simulink model "LUT_kidney_25"  (R2023b)
settings: Solver=FixedStepAuto  StartTime=0  StopTime=10.1  FixedStep=Timegap  RelTol=1e-3
model workspace (MAT data in the model file):
  T1_input = 1.34
(part 2 of 3)

== system LUT_kidney_25/If Action Subsystem6/If Action Subsystem1/If Action Subsystem6/If Action Subsystem4 ==
  In1 : Inport
  Action Port : ActionPort  ActionPortLabel=elseif( u1 >= 1.035)
  LUT 1.04RR : Lookup_n-D  NumberOfTableDimensions=1  BreakpointsForDimension1=[434.5226;535.5743;634.3365;733.4874;832.6376;931.7698;1030.887;1129.994;1229.093;1328.188;1427.279;1526.369;1625.457;1724.544;1823.63;1922.716;2021.797]  Table=[400;500;600;700;800;900;1000;1100;1200;1300;1400;1500;1600;1700;1800;1900;2000]  InternalRulePriority=Speed  RndMeth=Simplest
  Out1 : Outport
  wires:
  In1/1 -> LUT 1.04RR/1
  LUT 1.04RR/1 -> Out1/1

== system LUT_kidney_25/If Action Subsystem6/If Action Subsystem1/If Action Subsystem6/If Action Subsystem5 ==
  In1 : Inport
  Action Port : ActionPort  ActionPortLabel=elseif( u1 >= 1.055)
  LUT 1.06RR : Lookup_n-D  NumberOfTableDimensions=1  BreakpointsForDimension1=[434.2491;535.1556;633.7517;732.7193;831.6764;930.6091;1029.523;1128.423;1227.313;1326.197;1425.077;1523.953;1622.827;1721.7;1820.571;1919.441;2018.308]  Table=[400;500;600;700;800;900;1000;1100;1200;1300;1400;1500;1600;1700;1800;1900;2000]  InternalRulePriority=Speed  RndMeth=Simplest
  Out1 : Outport
  wires:
  In1/1 -> LUT 1.06RR/1
  LUT 1.06RR/1 -> Out1/1

== system LUT_kidney_25/If Action Subsystem6/If Action Subsystem1/If Action Subsystem6/If Action Subsystem6 ==
  In1 : Inport
  Action Port : ActionPort  ActionPortLabel=elseif( u1 >= 1.045)
  LUT 1.05RR : Lookup_n-D  NumberOfTableDimensions=1  BreakpointsForDimension1=[434.3843;535.3623;634.0403;733.0983;832.1508;931.1821;1030.196;1129.199;1228.192;1327.181;1426.165;1525.147;1624.126;1723.105;1822.083;1921.059;2020.032]  Table=[400;500;600;700;800;900;1000;1100;1200;1300;1400;1500;1600;1700;1800;1900;2000]  InternalRulePriority=Speed  RndMeth=Simplest
  Out1 : Outport
  wires:
  In1/1 -> LUT 1.05RR/1
  LUT 1.05RR/1 -> Out1/1

== system LUT_kidney_25/If Action Subsystem6/If Action Subsystem1/If Action Subsystem6/If Action Subsystem7 ==
  In1 : Inport
  Action Port : ActionPort  ActionPortLabel=elseif( u1 >= 1.065)
  LUT 1.07RR : Lookup_n-D  NumberOfTableDimensions=1  BreakpointsForDimension1=[434.1166;534.9541;633.4706;732.35;831.2139;930.0504;1028.866;1127.666;1226.455;1325.237;1424.014;1522.787;1621.558;1720.327;1819.094;1917.859;2016.622]  Table=[400;500;600;700;800;900;1000;1100;1200;1300;1400;1500;1600;1700;1800;1900;2000]  InternalRulePriority=Speed  RndMeth=Simplest
  Out1 : Outport
  wires:
  In1/1 -> LUT 1.07RR/1
  LUT 1.07RR/1 -> Out1/1

== system LUT_kidney_25/If Action Subsystem6/If Action Subsystem1/If Action Subsystem6/If Action Subsystem8 ==
  In1 : Inport
  Action Port : ActionPort  ActionPortLabel=elseif(u1 >= 1.075)
  LUT 1.08RR : Lookup_n-D  NumberOfTableDimensions=1  BreakpointsForDimension1=[433.987;534.7575;633.1966;731.9901;830.763;929.5054;1028.224;1126.927;1225.617;1324.299;1422.976;1521.648;1620.317;1718.984;1817.65;1916.313;2014.973]  Table=[400;500;600;700;800;900;1000;1100;1200;1300;1400;1500;1600;1700;1800;1900;2000]  InternalRulePriority=Speed  RndMeth=Simplest
  Out1 : Outport
  wires:
  In1/1 -> LUT 1.08RR/1
  LUT 1.08RR/1 -> Out1/1

== system LUT_kidney_25/If Action Subsystem6/If Action Subsystem1/If Action Subsystem6/If Action Subsystem9 ==
  In1 : Inport
  Action Port : ActionPort  ActionPortLabel=if(u1 >= 1.085)
  LUT 1.09RR : Lookup_n-D  NumberOfTableDimensions=1  BreakpointsForDimension1=[433.8599;534.5681;632.9294;731.6391;830.3233;928.9736;1027.598;1126.205;1224.799;1323.383;1421.962;1520.535;1619.105;1717.672;1816.237;1914.801;2013.361]  Table=[400;500;600;700;800;900;1000;1100;1200;1300;1400;1500;1600;1700;1800;1900;2000]  InternalRulePriority=Speed  RndMeth=Simplest
  Out1 : Outport
  wires:
  In1/1 -> LUT 1.09RR/1
  LUT 1.09RR/1 -> Out1/1

== system LUT_kidney_25/If Action Subsystem6/If Action Subsystem1/If Action Subsystem7/If Action Subsystem1 ==
  In1 : Inport
  Action Port : ActionPort  ActionPortLabel=elseif( u1 >= 1.215)
  LUT 1.22RR : Lookup_n-D  NumberOfTableDimensions=1  BreakpointsForDimension1=[432.4057;532.4278;629.9781;727.7664;825.4645;923.086;1020.653;1118.181;1215.681;1313.16;1410.624;1508.077;1605.521;1702.957;1800.388;1897.814;1995.235]  Table=[400;500;600;700;800;900;1000;1100;1200;1300;1400;1500;1600;1700;1800;1900;2000]  InternalRulePriority=Speed  RndMeth=Simplest
  Out1 : Outport
  wires:
  In1/1 -> LUT 1.22RR/1
  LUT 1.22RR/1 -> Out1/1

== system LUT_kidney_25/If Action Subsystem6/If Action Subsystem1/If Action Subsystem7/If Action Subsystem10 ==
  In1 : Inport
  Action Port : ActionPort  ActionPortLabel=elseif( u1 >= 1.205)
  LUT 1.21RR : Lookup_n-D  NumberOfTableDimensions=1  BreakpointsForDimension1=[432.5065;532.5721;630.1754;728.0248;825.789;923.48;1021.118;1118.72;1216.294;1313.849;1411.39;1508.919;1606.44;1703.953;1801.462;1898.966;1996.466]  Table=[400;500;600;700;800;900;1000;1100;1200;1300;1400;1500;1600;1700;1800;1900;2000]  InternalRulePriority=Speed  RndMeth=Simplest
  Out1 : Outport
  wires:
  In1/1 -> LUT 1.21RR/1
  LUT 1.21RR/1 -> Out1/1

== system LUT_kidney_25/If Action Subsystem6/If Action Subsystem1/If Action Subsystem7/If Action Subsystem2 ==
  In1 : Inport
  Action Port : ActionPort  ActionPortLabel=else
  LUT 1.20RR : Lookup_n-D  NumberOfTableDimensions=1  BreakpointsForDimension1=[432.6089;532.7193;630.3771;728.2891;826.1208;923.8827;1021.594;1119.27;1216.921;1314.553;1412.171;1509.778;1607.377;1704.97;1802.558;1900.141;1997.72]  Table=[400;500;600;700;800;900;1000;1100;1200;1300;1400;1500;1600;1700;1800;1900;2000]  InternalRulePriority=Speed  RndMeth=Simplest
  Out1 : Outport
  wires:
  In1/1 -> LUT 1.20RR/1
  LUT 1.20RR/1 -> Out1/1

== system LUT_kidney_25/If Action Subsystem6/If Action Subsystem1/If Action Subsystem7/If Action Subsystem3 ==
  In1 : Inport
  Action Port : ActionPort  ActionPortLabel=elseif( u1 >= 1.225)
  LUT 1.23RR : Lookup_n-D  NumberOfTableDimensions=1  BreakpointsForDimension1=[432.3064;532.2863;629.7849;727.5136;825.147;922.7006;1020.197;1117.653;1215.08;1312.485;1409.875;1507.252;1604.62;1701.98;1799.335;1896.684;1994.029]  Table=[400;500;600;700;800;900;1000;1100;1200;1300;1400;1500;1600;1700;1800;1900;2000]  InternalRulePriority=Speed  RndMeth=Simplest
  Out1 : Outport
  wires:
  In1/1 -> LUT 1.23RR/1
  LUT 1.23RR/1 -> Out1/1

== system LUT_kidney_25/If Action Subsystem6/If Action Subsystem1/If Action Subsystem7/If Action Subsystem4 ==
  In1 : Inport
  Action Port : ActionPort  ActionPortLabel=elseif( u1 >= 1.235)
  LUT 1.24RR : Lookup_n-D  NumberOfTableDimensions=1  BreakpointsForDimension1=[432.2086;532.1477;629.596;727.2663;824.8365;922.3235;1019.751;1117.136;1214.492;1311.824;1409.14;1506.444;1603.737;1701.023;1798.302;1895.576;1992.846]  Table=[400;500;600;700;800;900;1000;1100;1200;1300;1400;1500;1600;1700;1800;1900;2000]  InternalRulePriority=Speed  RndMeth=Simplest
  Out1 : Outport
  wires:
  In1/1 -> LUT 1.24RR/1
  LUT 1.24RR/1 -> Out1/1

== system LUT_kidney_25/If Action Subsystem6/If Action Subsystem1/If Action Subsystem7/If Action Subsystem5 ==
  In1 : Inport
  Action Port : ActionPort  ActionPortLabel=elseif( u1 >= 1.255)
  LUT 1.26RR : Lookup_n-D  NumberOfTableDimensions=1  BreakpointsForDimension1=[432.0174;531.8783;629.2298;726.7877;824.2353;921.5931;1018.887;1116.135;1213.351;1310.542;1407.715;1504.875;1602.023;1699.163;1796.297;1893.424;1990.547]  Table=[400;500;600;700;800;900;1000;1100;1200;1300;1400;1500;1600;1700;1800;1900;2000]  InternalRulePriority=Speed  RndMeth=Simplest
  Out1 : Outport
  wires:
  In1/1 -> LUT 1.26RR/1
  LUT 1.26RR/1 -> Out1/1

== system LUT_kidney_25/If Action Subsystem6/If Action Subsystem1/If Action Subsystem7/If Action Subsystem6 ==
  In1 : Inport
  Action Port : ActionPort  ActionPortLabel=elseif( u1 >= 1.245)
  LUT 1.25RR : Lookup_n-D  NumberOfTableDimensions=1  BreakpointsForDimension1=[432.1123;532.0117;629.411;727.0244;824.5326;921.9544;1019.314;1116.631;1213.915;1311.177;1408.421;1505.651;1602.872;1700.084;1797.29;1894.49;1991.685]  Table=[400;500;600;700;800;900;1000;1100;1200;1300;1400;1500;1600;1700;1800;1900;2000]  InternalRulePriority=Speed  RndMeth=Simplest
  Out1 : Outport
  wires:
  In1/1 -> LUT 1.25RR/1
  LUT 1.25RR/1 -> Out1/1

== system LUT_kidney_25/If Action Subsystem6/If Action Subsystem1/If Action Subsystem7/If Action Subsystem7 ==
  In1 : Inport
  Action Port : ActionPort  ActionPortLabel=elseif( u1 >= 1.265)
  LUT 1.27RR : Lookup_n-D  NumberOfTableDimensions=1  BreakpointsForDimension1=[431.9239;531.7475;629.0525;726.556;823.9443;921.2395;1018.468;1115.65;1212.798;1309.92;1407.024;1504.113;1601.191;1698.26;1795.322;1892.379;1989.43]  Table=[400;500;600;700;800;900;1000;1100;1200;1300;1400;1500;1600;1700;1800;1900;2000]  InternalRulePriority=Speed  RndMeth=Simplest
  Out1 : Outport
  wires:
  In1/1 -> LUT 1.27RR/1
  LUT 1.27RR/1 -> Out1/1

== system LUT_kidney_25/If Action Subsystem6/If Action Subsystem1/If Action Subsystem7/If Action Subsystem8 ==
  In1 : Inport
  Action Port : ActionPort  ActionPortLabel=elseif(u1 >= 1.275)
  LUT 1.28RR : Lookup_n-D  NumberOfTableDimensions=1  BreakpointsForDimension1=[431.8317;531.6191;628.8788;726.3292;823.6595;920.8933;1018.058;1115.175;1212.256;1309.311;1406.346;1503.366;1600.375;1697.375;1794.367;1891.353;1988.334]  Table=[400;500;600;700;800;900;1000;1100;1200;1300;1400;1500;1600;1700;1800;1900;2000]  InternalRulePriority=Speed  RndMeth=Simplest
  Out1 : Outport
  wires:
  In1/1 -> LUT 1.28RR/1
  LUT 1.28RR/1 -> Out1/1

== system LUT_kidney_25/If Action Subsystem6/If Action Subsystem1/If Action Subsystem7/If Action Subsystem9 ==
  In1 : Inport
  Action Port : ActionPort  ActionPortLabel=if(u1 >= 1.285)
  LUT 1.29RR : Lookup_n-D  NumberOfTableDimensions=1  BreakpointsForDimension1=[431.7409;531.4931;628.7087;726.1072;823.3807;920.5544;1017.657;1114.709;1211.725;1308.713;1405.681;1502.634;1599.575;1696.506;1793.429;1890.346;1987.258]  Table=[400;500;600;700;800;900;1000;1100;1200;1300;1400;1500;1600;1700;1800;1900;2000]  InternalRulePriority=Speed  RndMeth=Simplest
  Out1 : Outport
  wires:
  In1/1 -> LUT 1.29RR/1
  LUT 1.29RR/1 -> Out1/1

== system LUT_kidney_25/If Action Subsystem6/If Action Subsystem1/If Action Subsystem8/If Action Subsystem1 ==
  In1 : Inport
  Action Port : ActionPort  ActionPortLabel=elseif( u1 >= 1.315)
  LUT 1.32RR : Lookup_n-D  NumberOfTableDimensions=1  BreakpointsForDimension1=[431.4756;531.1287;628.2187;725.4687;822.5789;919.5791;1016.501;1113.368;1210.194;1306.99;1403.764;1500.521;1597.264;1693.997;1790.721;1887.438;1984.149]  Table=[400;500;600;700;800;900;1000;1100;1200;1300;1400;1500;1600;1700;1800;1900;2000]  InternalRulePriority=Speed  RndMeth=Simplest
  Out1 : Outport
  wires:
  In1/1 -> LUT 1.32RR/1
  LUT 1.32RR/1 -> Out1/1

== system LUT_kidney_25/If Action Subsystem6/If Action Subsystem1/If Action Subsystem8/If Action Subsystem10 ==
  In1 : Inport
  Action Port : ActionPort  ActionPortLabel=elseif( u1 >= 1.305)
  LUT 1.31RR : Lookup_n-D  NumberOfTableDimensions=1  BreakpointsForDimension1=[431.5628;531.248;628.3787;725.6771;822.8406;919.8974;1016.879;1113.806;1210.694;1307.553;1404.391;1501.212;1598.02;1694.817;1791.607;1888.389;1985.166]  Table=[400;500;600;700;800;900;1000;1100;1200;1300;1400;1500;1600;1700;1800;1900;2000]  InternalRulePriority=Speed  RndMeth=Simplest
  Out1 : Outport
  wires:
  In1/1 -> LUT 1.31RR/1
  LUT 1.31RR/1 -> Out1/1

== system LUT_kidney_25/If Action Subsystem6/If Action Subsystem1/If Action Subsystem8/If Action Subsystem2 ==
  In1 : Inport
  Action Port : ActionPort  ActionPortLabel=else
  LUT 1.30RR : Lookup_n-D  NumberOfTableDimensions=1  BreakpointsForDimension1=[431.6512;531.3694;628.542;725.8899;823.1078;920.2225;1017.264;1114.253;1211.204;1308.127;1405.03;1501.916;1598.79;1695.654;1792.509;1889.359;1986.202]  Table=[400;500;600;700;800;900;1000;1100;1200;1300;1400;1500;1600;1700;1800;1900;2000]  InternalRulePriority=Speed  RndMeth=Simplest
  Out1 : Outport
  wires:
  In1/1 -> LUT 1.30RR/1
  LUT 1.30RR/1 -> Out1/1

== system LUT_kidney_25/If Action Subsystem6/If Action Subsystem1/If Action Subsystem8/If Action Subsystem3 ==
  In1 : Inport
  Action Port : ActionPort  ActionPortLabel=elseif( u1 >= 1.325)
  LUT 1.33RR : Lookup_n-D  NumberOfTableDimensions=1  BreakpointsForDimension1=[431.3895;531.0116;628.0619;725.2646;822.3226;919.2673;1016.131;1112.938;1209.703;1306.438;1403.149;1499.843;1596.523;1693.191;1789.851;1886.503;1983.15]  Table=[400;500;600;700;800;900;1000;1100;1200;1300;1400;1500;1600;1700;1800;1900;2000]  InternalRulePriority=Speed  RndMeth=Simplest
  Out1 : Outport
  wires:
  In1/1 -> LUT 1.33RR/1
  LUT 1.33RR/1 -> Out1/1

== system LUT_kidney_25/If Action Subsystem6/If Action Subsystem1/If Action Subsystem8/If Action Subsystem4 ==
  In1 : Inport
  Action Port : ActionPort  ActionPortLabel=elseif( u1 >= 1.335)
  LUT 1.34RR : Lookup_n-D  NumberOfTableDimensions=1  BreakpointsForDimension1=[431.3046;530.8966;627.9082;725.0647;822.0716;918.9618;1015.769;1112.517;1209.223;1305.897;1402.546;1499.178;1595.795;1692.401;1788.997;1885.586;1982.169]  Table=[400;500;600;700;800;900;1000;1100;1200;1300;1400;1500;1600;1700;1800;1900;2000]  InternalRulePriority=Speed  RndMeth=Simplest
  Out1 : Outport
  wires:
  In1/1 -> LUT 1.34RR/1
  LUT 1.34RR/1 -> Out1/1

== system LUT_kidney_25/If Action Subsystem6/If Action Subsystem1/If Action Subsystem8/If Action Subsystem5 ==
  In1 : Inport
  Action Port : ActionPort  ActionPortLabel=elseif( u1 >= 1.355)
  LUT 1.36RR : Lookup_n-D  NumberOfTableDimensions=1  BreakpointsForDimension1=[431.138;530.6725;627.6097;724.6771;821.585;918.3694;1015.066;1111.7;1208.289;1304.845;1401.375;1497.885;1594.38;1690.863;1787.336;1883.801;1980.259]  Table=[400;500;600;700;800;900;1000;1100;1200;1300;1400;1500;1600;1700;1800;1900;2000]  InternalRulePriority=Speed  RndMeth=Simplest
  Out1 : Outport
  wires:
  In1/1 -> LUT 1.36RR/1
  LUT 1.36RR/1 -> Out1/1

== system LUT_kidney_25/If Action Subsystem6/If Action Subsystem1/If Action Subsystem8/If Action Subsystem6 ==
  In1 : Inport
  Action Port : ActionPort  ActionPortLabel=elseif( u1 >= 1.345)
  LUT 1.35RR : Lookup_n-D  NumberOfTableDimensions=1  BreakpointsForDimension1=[431.2207;530.7835;627.7575;724.8689;821.8258;918.6626;1015.414;1112.105;1208.752;1305.366;1401.955;1498.525;1595.081;1691.625;1788.159;1884.686;1981.205]  Table=[400;500;600;700;800;900;1000;1100;1200;1300;1400;1500;1600;1700;1800;1900;2000]  InternalRulePriority=Speed  RndMeth=Simplest
  Out1 : Outport
  wires:
  In1/1 -> LUT 1.35RR/1
  LUT 1.35RR/1 -> Out1/1

== system LUT_kidney_25/If Action Subsystem6/If Action Subsystem1/If Action Subsystem8/If Action Subsystem7 ==
  In1 : Inport
  Action Port : ActionPort  ActionPortLabel=elseif( u1 >= 1.365)
  LUT 1.37RR : Lookup_n-D  NumberOfTableDimensions=1  BreakpointsForDimension1=[431.0562;530.5633;627.4649;724.4891;821.3491;918.0821;1014.725;1111.304;1207.836;1304.334;1400.805;1497.256;1593.692;1690.115;1786.528;1882.932;1979.33]  Table=[400;500;600;700;800;900;1000;1100;1200;1300;1400;1500;1600;1700;1800;1900;2000]  InternalRulePriority=Speed  RndMeth=Simplest
  Out1 : Outport
  wires:
  In1/1 -> LUT 1.37RR/1
  LUT 1.37RR/1 -> Out1/1

== system LUT_kidney_25/If Action Subsystem6/If Action Subsystem1/If Action Subsystem8/If Action Subsystem8 ==
  In1 : Inport
  Action Port : ActionPort  ActionPortLabel=elseif(u1 >= 1.375)
  LUT 1.38RR : Lookup_n-D  NumberOfTableDimensions=1  BreakpointsForDimension1=[430.9755;530.4561;627.3228;724.305;821.1179;917.8006;1014.391;1110.915;1207.392;1303.832;1400.246;1496.64;1593.017;1689.381;1785.734;1882.079;1978.417]  Table=[400;500;600;700;800;900;1000;1100;1200;1300;1400;1500;1600;1700;1800;1900;2000]  InternalRulePriority=Speed  RndMeth=Simplest
  Out1 : Outport
  wires:
  In1/1 -> LUT 1.38RR/1
  LUT 1.38RR/1 -> Out1/1

== system LUT_kidney_25/If Action Subsystem6/If Action Subsystem1/If Action Subsystem8/If Action Subsystem9 ==
  In1 : Inport
  Action Port : ActionPort  ActionPortLabel=if(u1 >= 1.385)
  LUT 1.39RR : Lookup_n-D  NumberOfTableDimensions=1  BreakpointsForDimension1=[430.8958;530.3506;627.1835;724.1245;820.8914;917.5247;1014.063;1110.534;1206.956;1303.341;1399.698;1496.034;1592.353;1688.659;1784.955;1881.241;1977.521]  Table=[400;500;600;700;800;900;1000;1100;1200;1300;1400;1500;1600;1700;1800;1900;2000]  InternalRulePriority=Speed  RndMeth=Simplest
  Out1 : Outport
  wires:
  In1/1 -> LUT 1.39RR/1
  LUT 1.39RR/1 -> Out1/1

== system LUT_kidney_25/If Action Subsystem6/If Action Subsystem1/If Action Subsystem9/If Action Subsystem1 ==
  In1 : Inport
  Action Port : ActionPort  ActionPortLabel=elseif( u1 >= 1.415)
  LUT 1.42RR : Lookup_n-D  NumberOfTableDimensions=1  BreakpointsForDimension1=[430.6624;530.0447;626.7812;723.6044;820.2389;916.7296;1013.118;1109.434;1205.697;1301.92;1398.113;1494.283;1590.435;1686.572;1782.698;1878.814;1974.923]  Table=[400;500;600;700;800;900;1000;1100;1200;1300;1400;1500;1600;1700;1800;1900;2000]  InternalRulePriority=Speed  RndMeth=Simplest
  Out1 : Outport
  wires:
  In1/1 -> LUT 1.42RR/1
  LUT 1.42RR/1 -> Out1/1

== system LUT_kidney_25/If Action Subsystem6/If Action Subsystem1/If Action Subsystem9/If Action Subsystem10 ==
  In1 : Inport
  Action Port : ActionPort  ActionPortLabel=elseif( u1 >= 1.405)
  LUT 1.41RR : Lookup_n-D  NumberOfTableDimensions=1  BreakpointsForDimension1=[430.7393;530.1449;626.9128;723.7743;820.452;916.9894;1013.427;1109.794;1206.108;1302.384;1398.631;1494.856;1591.063;1687.256;1783.437;1879.609;1975.774]  Table=[400;500;600;700;800;900;1000;1100;1200;1300;1400;1500;1600;1700;1800;1900;2000]  InternalRulePriority=Speed  RndMeth=Simplest
  Out1 : Outport
  wires:
  In1/1 -> LUT 1.41RR/1
  LUT 1.41RR/1 -> Out1/1

== system LUT_kidney_25/If Action Subsystem6/If Action Subsystem1/If Action Subsystem9/If Action Subsystem2 ==
  In1 : Inport
  Action Port : ActionPort  ActionPortLabel=else
  LUT 1.40RR : Lookup_n-D  NumberOfTableDimensions=1  BreakpointsForDimension1=[430.8171;530.2469;627.0468;723.9476;820.6695;917.2544;1013.742;1110.16;1206.528;1302.858;1399.16;1495.44;1591.702;1687.951;1784.189;1880.418;1976.639]  Table=[400;500;600;700;800;900;1000;1100;1200;1300;1400;1500;1600;1700;1800;1900;2000]  InternalRulePriority=Speed  RndMeth=Simplest
  Out1 : Outport
  wires:
  In1/1 -> LUT 1.40RR/1
  LUT 1.40RR/1 -> Out1/1

== system LUT_kidney_25/If Action Subsystem6/If Action Subsystem1/If Action Subsystem9/If Action Subsystem3 ==
  In1 : Inport
  Action Port : ActionPort  ActionPortLabel=elseif( u1 >= 1.425)
  LUT 1.43RR : Lookup_n-D  NumberOfTableDimensions=1  BreakpointsForDimension1=[430.5865;529.946;626.6522;723.4378;820.03;916.475;1012.816;1109.081;1205.293;1301.464;1397.604;1493.72;1589.818;1685.901;1781.972;1878.034;1974.087]  Table=[400;500;600;700;800;900;1000;1100;1200;1300;1400;1500;1600;1700;1800;1900;2000]  InternalRulePriority=Speed  RndMeth=Simplest
  Out1 : Outport
  wires:
  In1/1 -> LUT 1.43RR/1
  LUT 1.43RR/1 -> Out1/1

== system LUT_kidney_25/If Action Subsystem6/If Action Subsystem1/If Action Subsystem9/If Action Subsystem4 ==
  In1 : Inport
  Action Port : ActionPort  ActionPortLabel=elseif( u1 >= 1.435)
  LUT 1.44RR : Lookup_n-D  NumberOfTableDimensions=1  BreakpointsForDimension1=[430.5114;529.849;626.5256;723.2745;819.8252;916.2254;1012.519;1108.735;1204.896;1301.016;1397.104;1493.168;1589.213;1685.242;1781.259;1877.266;1973.265]  Table=[400;500;600;700;800;900;1000;1100;1200;1300;1400;1500;1600;1700;1800;1900;2000]  InternalRulePriority=Speed  RndMeth=Simplest
  Out1 : Outport
  wires:
  In1/1 -> LUT 1.44RR/1
  LUT 1.44RR/1 -> Out1/1

== system LUT_kidney_25/If Action Subsystem6/If Action Subsystem1/If Action Subsystem9/If Action Subsystem5 ==
  In1 : Inport
  Action Port : ActionPort  ActionPortLabel=elseif( u1 >= 1.455)
  LUT 1.46RR : Lookup_n-D  NumberOfTableDimensions=1  BreakpointsForDimension1=[430.3639;529.6596;626.2793;722.9574;819.4277;915.7408;1011.942;1108.063;1204.126;1300.145;1396.132;1492.092;1588.033;1683.958;1779.869;1875.771;1971.663]  Table=[400;500;600;700;800;900;1000;1100;1200;1300;1400;1500;1600;1700;1800;1900;2000]  InternalRulePriority=Speed  RndMeth=Simplest
  Out1 : Outport
  wires:
  In1/1 -> LUT 1.46RR/1
  LUT 1.46RR/1 -> Out1/1

== system LUT_kidney_25/If Action Subsystem6/If Action Subsystem1/If Action Subsystem9/If Action Subsystem6 ==
  In1 : Inport
  Action Port : ActionPort  ActionPortLabel=elseif( u1 >= 1.445)
  LUT 1.45RR : Lookup_n-D  NumberOfTableDimensions=1  BreakpointsForDimension1=[430.4372;529.7535;626.4013;723.1144;819.6245;915.9807;1012.228;1108.396;1204.508;1300.577;1396.613;1492.625;1588.618;1684.594;1780.558;1876.512;1972.457]  Table=[400;500;600;700;800;900;1000;1100;1200;1300;1400;1500;1600;1700;1800;1900;2000]  InternalRulePriority=Speed  RndMeth=Simplest
  Out1 : Outport
  wires:
  In1/1 -> LUT 1.45RR/1
  LUT 1.45RR/1 -> Out1/1

== system LUT_kidney_25/If Action Subsystem6/If Action Subsystem1/If Action Subsystem9/If Action Subsystem7 ==
  In1 : Inport
  Action Port : ActionPort  ActionPortLabel=elseif( u1 >= 1.465)
  LUT 1.47RR : Lookup_n-D  NumberOfTableDimensions=1  BreakpointsForDimension1=[430.2914;529.5672;626.1596;722.8035;819.2349;915.5055;1011.662;1107.737;1203.752;1299.722;1395.659;1491.569;1587.459;1683.332;1779.193;1875.042;1970.882]  Table=[400;500;600;700;800;900;1000;1100;1200;1300;1400;1500;1600;1700;1800;1900;2000]  InternalRulePriority=Speed  RndMeth=Simplest
  Out1 : Outport
  wires:
  In1/1 -> LUT 1.47RR/1
  LUT 1.47RR/1 -> Out1/1

== system LUT_kidney_25/If Action Subsystem6/If Action Subsystem1/If Action Subsystem9/If Action Subsystem8 ==
  In1 : Inport
  Action Port : ActionPort  ActionPortLabel=elseif(u1 >= 1.475)
  LUT 1.48RR : Lookup_n-D  NumberOfTableDimensions=1  BreakpointsForDimension1=[430.2197;529.4762;626.042;722.6526;819.0457;915.2748;1011.387;1107.416;1203.384;1299.306;1395.194;1491.055;1586.895;1682.718;1778.527;1874.326;1970.115]  Table=[400;500;600;700;800;900;1000;1100;1200;1300;1400;1500;1600;1700;1800;1900;2000]  InternalRulePriority=Speed  RndMeth=Simplest
  Out1 : Outport
  wires:
  In1/1 -> LUT 1.48RR/1
  LUT 1.48RR/1 -> Out1/1

== system LUT_kidney_25/If Action Subsystem6/If Action Subsystem1/If Action Subsystem9/If Action Subsystem9 ==
  In1 : Inport
  Action Port : ActionPort  ActionPortLabel=if(u1 >= 1.485)
  LUT 1.49RR : Lookup_n-D  NumberOfTableDimensions=1  BreakpointsForDimension1=[430.1488;529.3866;625.9267;722.5045;818.8603;915.0486;1011.118;1107.102;1203.023;1298.898;1394.738;1490.55;1586.34;1682.114;1777.873;1873.621;1969.36]  Table=[400;500;600;700;800;900;1000;1100;1200;1300;1400;1500;1600;1700;1800;1900;2000]  InternalRulePriority=Speed  RndMeth=Simplest
  Out1 : Outport
  wires:
  In1/1 -> LUT 1.49RR/1
  LUT 1.49RR/1 -> Out1/1

== system LUT_kidney_25/If Action Subsystem6/If Action Subsystem2/If Action Subsystem5/If Action Subsystem1 ==
  In1 : Inport
  Action Port : ActionPort  ActionPortLabel=elseif( u1 >= 1.615)
  LUT 1.62RR : Lookup_n-D  NumberOfTableDimensions=1  BreakpointsForDimension1=[429.2939;528.3389;624.6015;720.8179;816.7518;912.4744;1008.046;1103.509;1198.891;1294.214;1389.49;1484.731;1579.943;1675.133;1770.305;1865.462;1960.606]  Table=[400;500;600;700;800;900;1000;1100;1200;1300;1400;1500;1600;1700;1800;1900;2000]  InternalRulePriority=Speed  RndMeth=Simplest
  Out1 : Outport
  wires:
  In1/1 -> LUT 1.62RR/1
  LUT 1.62RR/1 -> Out1/1

== system LUT_kidney_25/If Action Subsystem6/If Action Subsystem2/If Action Subsystem5/If Action Subsystem10 ==
  In1 : Inport
  Action Port : ActionPort  ActionPortLabel=elseif( u1>= 1.605)
  LUT 1.61RR : Lookup_n-D  NumberOfTableDimensions=1  BreakpointsForDimension1=[429.3556;528.4125;624.6929;720.9334;816.8958;912.6504;1008.256;1103.755;1199.175;1294.536;1389.852;1485.133;1580.387;1675.618;1770.831;1866.029;1961.215]  Table=[400;500;600;700;800;900;1000;1100;1200;1300;1400;1500;1600;1700;1800;1900;2000]  InternalRulePriority=Speed  RndMeth=Simplest
  Out1 : Outport
  wires:
  In1/1 -> LUT 1.61RR/1
  LUT 1.61RR/1 -> Out1/1

== system LUT_kidney_25/If Action Subsystem6/If Action Subsystem2/If Action Subsystem5/If Action Subsystem2 ==
  In1 : Inport
  Action Port : ActionPort  ActionPortLabel=else
  LUT 1.60RR : Lookup_n-D  NumberOfTableDimensions=1  BreakpointsForDimension1=[429.4179;528.4872;624.786;721.0511;817.0427;912.8298;1008.471;1104.007;1199.465;1294.865;1390.221;1485.543;1580.837;1676.11;1771.365;1866.606;1961.835]  Table=[400;500;600;700;800;900;1000;1100;1200;1300;1400;1500;1600;1700;1800;1900;2000]  InternalRulePriority=Speed  RndMeth=Simplest
  Out1 : Outport
  wires:
  In1/1 -> LUT 1.60RR/1
  LUT 1.60RR/1 -> Out1/1

== system LUT_kidney_25/If Action Subsystem6/If Action Subsystem2/If Action Subsystem5/If Action Subsystem3 ==
  In1 : Inport
  Action Port : ActionPort  ActionPortLabel=elseif( u1 >= 1.625)
  LUT 1.63RR : Lookup_n-D  NumberOfTableDimensions=1  BreakpointsForDimension1=[429.2328;528.2663;624.5116;720.7045;816.6104;912.3017;1007.84;1103.267;1198.612;1293.896;1389.134;1484.335;1579.507;1674.657;1769.788;1864.903;1960.006]  Table=[400;500;600;700;800;900;1000;1100;1200;1300;1400;1500;1600;1700;1800;1900;2000]  InternalRulePriority=Speed  RndMeth=Simplest
  Out1 : Outport
  wires:
  In1/1 -> LUT 1.63RR/1
  LUT 1.63RR/1 -> Out1/1

== system LUT_kidney_25/If Action Subsystem6/If Action Subsystem2/If Action Subsystem5/If Action Subsystem4 ==
  In1 : Inport
  Action Port : ActionPort  ActionPortLabel=elseif( u1 >= 1.635)
  LUT 1.64RR : Lookup_n-D  NumberOfTableDimensions=1  BreakpointsForDimension1=[429.1723;528.1948;624.4232;720.5933;816.4718;912.1323;1007.637;1103.029;1198.338;1293.585;1388.784;1483.946;1579.079;1674.188;1769.279;1864.354;1959.416]  Table=[400;500;600;700;800;900;1000;1100;1200;1300;1400;1500;1600;1700;1800;1900;2000]  InternalRulePriority=Speed  RndMeth=Simplest
  Out1 : Outport
  wires:
  In1/1 -> LUT 1.64RR/1
  LUT 1.64RR/1 -> Out1/1

== system LUT_kidney_25/If Action Subsystem6/If Action Subsystem2/If Action Subsystem5/If Action Subsystem5 ==
  In1 : Inport
  Action Port : ActionPort  ActionPortLabel=elseif( u1 >= 1.655)
  LUT 1.66RR : Lookup_n-D  NumberOfTableDimensions=1  BreakpointsForDimension1=[429.0532;528.0547;624.251;720.3769;816.2023;911.803;1007.243;1102.566;1197.804;1292.977;1388.102;1483.187;1578.243;1673.274;1768.285;1863.281;1958.262]  Table=[400;500;600;700;800;900;1000;1100;1200;1300;1400;1500;1600;1700;1800;1900;2000]  InternalRulePriority=Speed  RndMeth=Simplest
  Out1 : Outport
  wires:
  In1/1 -> LUT 1.66RR/1
  LUT 1.66RR/1 -> Out1/1

== system LUT_kidney_25/If Action Subsystem6/If Action Subsystem2/If Action Subsystem5/If Action Subsystem6 ==
  In1 : Inport
  Action Port : ActionPort  ActionPortLabel=elseif( u1 >= 1.645)
  LUT 1.65RR : Lookup_n-D  NumberOfTableDimensions=1  BreakpointsForDimension1=[429.1125;528.1243;624.3363;720.4841;816.3357;911.9661;1007.438;1102.795;1198.069;1293.278;1388.44;1483.563;1578.657;1673.727;1768.778;1863.813;1958.834]  Table=[400;500;600;700;800;900;1000;1100;1200;1300;1400;1500;1600;1700;1800;1900;2000]  InternalRulePriority=Speed  RndMeth=Simplest
  Out1 : Outport
  wires:
  In1/1 -> LUT 1.65RR/1
  LUT 1.65RR/1 -> Out1/1

== system LUT_kidney_25/If Action Subsystem6/If Action Subsystem2/If Action Subsystem5/If Action Subsystem7 ==
  In1 : Inport
  Action Port : ActionPort  ActionPortLabel=elseif( u1 >= 1.665)
  LUT 1.67RR : Lookup_n-D  NumberOfTableDimensions=1  BreakpointsForDimension1=[428.9945;527.9862;624.167;720.2717;816.0713;911.643;1007.051;1102.341;1197.544;1292.682;1387.769;1482.818;1577.835;1672.828;1767.801;1862.757;1957.699]  Table=[400;500;600;700;800;900;1000;1100;1200;1300;1400;1500;1600;1700;1800;1900;2000]  InternalRulePriority=Speed  RndMeth=Simplest
  Out1 : Outport
  wires:
  In1/1 -> LUT 1.67RR/1
  LUT 1.67RR/1 -> Out1/1

== system LUT_kidney_25/If Action Subsystem6/If Action Subsystem2/If Action Subsystem5/If Action Subsystem8 ==
  In1 : Inport
  Action Port : ActionPort  ActionPortLabel=elseif(u1 >= 1.675)
  LUT 1.68RR : Lookup_n-D  NumberOfTableDimensions=1  BreakpointsForDimension1=[428.9364;527.9185;624.0845;720.1684;815.9428;911.486;1006.863;1102.121;1197.289;1292.391;1387.442;1482.454;1577.434;1672.389;1767.324;1862.241;1957.145]  Table=[400;500;600;700;800;900;1000;1100;1200;1300;1400;1500;1600;1700;1800;1900;2000]  InternalRulePriority=Speed  RndMeth=Simplest
  Out1 : Outport
  wires:
  In1/1 -> LUT 1.68RR/1
  LUT 1.68RR/1 -> Out1/1

== system LUT_kidney_25/If Action Subsystem6/If Action Subsystem2/If Action Subsystem5/If Action Subsystem9 ==
  In1 : Inport
  Action Port : ActionPort  ActionPortLabel=if(u1 >= 1.685)
  LUT 1.69RR : Lookup_n-D  NumberOfTableDimensions=1  BreakpointsForDimension1=[428.8789;527.8519;624.0034;720.067;815.8168;911.3319;1006.679;1101.904;1197.039;1292.106;1387.121;1482.096;1577.04;1671.957;1766.854;1861.734;1956.6]  Table=[400;500;600;700;800;900;1000;1100;1200;1300;1400;1500;1600;1700;1800;1900;2000]  InternalRulePriority=Speed  RndMeth=Simplest
  Out1 : Outport
  wires:
  In1/1 -> LUT 1.69RR/1
  LUT 1.69RR/1 -> Out1/1

== system LUT_kidney_25/If Action Subsystem6/If Action Subsystem2/If Action Subsystem6/If Action Subsystem1 ==
  In1 : Inport
  Action Port : ActionPort  ActionPortLabel=elseif( u1 >= 1.515)
  LUT 1.52RR : Lookup_n-D  NumberOfTableDimensions=1  BreakpointsForDimension1=[429.9408;529.1262;625.5929;722.0773;818.3254;914.396;1010.34;1106.193;1201.98;1297.718;1393.417;1489.087;1584.735;1680.363;1775.977;1871.579;1967.17]  Table=[400;500;600;700;800;900;1000;1100;1200;1300;1400;1500;1600;1700;1800;1900;2000]  InternalRulePriority=Speed  RndMeth=Simplest
  Out1 : Outport
  wires:
  In1/1 -> LUT 1.52RR/1
  LUT 1.52RR/1 -> Out1/1

== system LUT_kidney_25/If Action Subsystem6/If Action Subsystem2/If Action Subsystem6/If Action Subsystem10 ==
  In1 : Inport
  Action Port : ActionPort  ActionPortLabel=elseif( u1 >= 1.505)
  LUT 1.51RR : Lookup_n-D  NumberOfTableDimensions=1  BreakpointsForDimension1=[430.0094;529.2117;625.7021;722.217;818.5002;914.6093;1010.594;1106.491;1202.322;1298.104;1393.849;1489.566;1585.261;1680.937;1776.599;1872.248;1967.888]  Table=[400;500;600;700;800;900;1000;1100;1200;1300;1400;1500;1600;1700;1800;1900;2000]  InternalRulePriority=Speed  RndMeth=Simplest
  Out1 : Outport
  wires:
  In1/1 -> LUT 1.51RR/1
  LUT 1.51RR/1 -> Out1/1

== system LUT_kidney_25/If Action Subsystem6/If Action Subsystem2/If Action Subsystem6/If Action Subsystem2 ==
  In1 : Inport
  Action Port : ActionPort  ActionPortLabel=else
  LUT 1.50RR : Lookup_n-D  NumberOfTableDimensions=1  BreakpointsForDimension1=[430.0787;529.2985;625.8134;722.3594;818.6785;914.8268;1010.854;1106.793;1202.669;1298.497;1394.29;1490.054;1585.796;1681.52;1777.23;1872.929;1968.618]  Table=[400;500;600;700;800;900;1000;1100;1200;1300;1400;1500;1600;1700;1800;1900;2000]  InternalRulePriority=Speed  RndMeth=Simplest
  Out1 : Outport
  wires:
  In1/1 -> LUT 1.50RR/1
  LUT 1.50RR/1 -> Out1/1

== system LUT_kidney_25/If Action Subsystem6/If Action Subsystem2/If Action Subsystem6/If Action Subsystem3 ==
  In1 : Inport
  Action Port : ActionPort  ActionPortLabel=elseif( u1 >= 1.525)
  LUT 1.53RR : Lookup_n-D  NumberOfTableDimensions=1  BreakpointsForDimension1=[429.873;529.0421;625.4856;721.9403;818.154;914.1867;1010.091;1105.902;1201.645;1297.338;1392.992;1488.617;1584.218;1679.8;1775.366;1870.921;1966.465]  Table=[400;500;600;700;800;900;1000;1100;1200;1300;1400;1500;1600;1700;1800;1900;2000]  InternalRulePriority=Speed  RndMeth=Simplest
  Out1 : Outport
  wires:
  In1/1 -> LUT 1.53RR/1
  LUT 1.53RR/1 -> Out1/1

== system LUT_kidney_25/If Action Subsystem6/If Action Subsystem2/If Action Subsystem6/If Action Subsystem4 ==
  In1 : Inport
  Action Port : ActionPort  ActionPortLabel=elseif( u1 >= 1.535)
  LUT 1.54RR : Lookup_n-D  NumberOfTableDimensions=1  BreakpointsForDimension1=[429.8059;528.9592;625.3803;721.8059;817.9859;913.9815;1009.846;1105.616;1201.316;1296.966;1392.575;1488.154;1583.71;1679.245;1774.766;1870.273;1965.77]  Table=[400;500;600;700;800;900;1000;1100;1200;1300;1400;1500;1600;1700;1800;1900;2000]  InternalRulePriority=Speed  RndMeth=Simplest
  Out1 : Outport
  wires:
  In1/1 -> LUT 1.54RR/1
  LUT 1.54RR/1 -> Out1/1

== system LUT_kidney_25/If Action Subsystem6/If Action Subsystem2/If Action Subsystem6/If Action Subsystem5 ==
  In1 : Inport
  Action Port : ActionPort  ActionPortLabel=elseif( u1 >= 1.555)
  LUT 1.56RR : Lookup_n-D  NumberOfTableDimensions=1  BreakpointsForDimension1=[429.6738;528.7972;625.1751;721.5446;817.6592;913.5827;1009.37;1105.059;1200.677;1296.24;1391.763;1487.254;1582.719;1678.165;1773.594;1869.01;1964.415]  Table=[400;500;600;700;800;900;1000;1100;1200;1300;1400;1500;1600;1700;1800;1900;2000]  InternalRulePriority=Speed  RndMeth=Simplest
  Out1 : Outport
  wires:
  In1/1 -> LUT 1.56RR/1
  LUT 1.56RR/1 -> Out1/1

== system LUT_kidney_25/If Action Subsystem6/If Action Subsystem2/If Action Subsystem6/If Action Subsystem6 ==
  In1 : Inport
  Action Port : ActionPort  ActionPortLabel=elseif( u1 >= 1.545)
  LUT 1.55RR : Lookup_n-D  NumberOfTableDimensions=1  BreakpointsForDimension1=[429.7395;528.8776;625.2768;721.674;817.821;913.7802;1009.606;1105.335;1200.994;1296.6;1392.165;1487.7;1583.21;1678.701;1774.175;1869.637;1965.087]  Table=[400;500;600;700;800;900;1000;1100;1200;1300;1400;1500;1600;1700;1800;1900;2000]  InternalRulePriority=Speed  RndMeth=Simplest
  Out1 : Outport
  wires:
  In1/1 -> LUT 1.55RR/1
  LUT 1.55RR/1 -> Out1/1

== system LUT_kidney_25/If Action Subsystem6/If Action Subsystem2/If Action Subsystem6/If Action Subsystem7 ==
  In1 : Inport
  Action Port : ActionPort  ActionPortLabel=elseif( u1 >= 1.565)
  LUT 1.57RR : Lookup_n-D  NumberOfTableDimensions=1  BreakpointsForDimension1=[429.6088;528.7179;625.0752;721.4177;817.5006;913.389;1009.139;1104.789;1200.365;1295.887;1391.367;1486.815;1582.237;1677.638;1773.023;1868.394;1963.755]  Table=[400;500;600;700;800;900;1000;1100;1200;1300;1400;1500;1600;1700;1800;1900;2000]  InternalRulePriority=Speed  RndMeth=Simplest
  Out1 : Outport
  wires:
  In1/1 -> LUT 1.57RR/1
  LUT 1.57RR/1 -> Out1/1

== system LUT_kidney_25/If Action Subsystem6/If Action Subsystem2/If Action Subsystem6/If Action Subsystem8 ==
  In1 : Inport
  Action Port : ActionPort  ActionPortLabel=elseif(u1 >= 1.575)
  LUT 1.58RR : Lookup_n-D  NumberOfTableDimensions=1  BreakpointsForDimension1=[429.5445;528.6399;624.9771;721.2932;817.345;913.199;1008.912;1104.523;1200.06;1295.54;1390.978;1486.383;1581.762;1677.12;1772.461;1867.789;1963.104]  Table=[400;500;600;700;800;900;1000;1100;1200;1300;1400;1500;1600;1700;1800;1900;2000]  InternalRulePriority=Speed  RndMeth=Simplest
  Out1 : Outport
  wires:
  In1/1 -> LUT 1.58RR/1
  LUT 1.58RR/1 -> Out1/1

== system LUT_kidney_25/If Action Subsystem6/If Action Subsystem2/If Action Subsystem6/If Action Subsystem9 ==
  In1 : Inport
  Action Port : ActionPort  ActionPortLabel=if(u1 >= 1.585)
  LUT 1.59RR : Lookup_n-D  NumberOfTableDimensions=1  BreakpointsForDimension1=[429.4809;528.563;624.8807;721.171;817.1924;913.0127;1008.689;1104.262;1199.76;1295.2;1390.597;1485.96;1581.296;1676.611;1771.909;1867.193;1962.464]  Table=[400;500;600;700;800;900;1000;1100;1200;1300;1400;1500;1600;1700;1800;1900;2000]  InternalRulePriority=Speed  RndMeth=Simplest
  Out1 : Outport
  wires:
  In1/1 -> LUT 1.59RR/1
  LUT 1.59RR/1 -> Out1/1

== system LUT_kidney_25/If Action Subsystem6/If Action Subsystem2/If Action Subsystem7/If Action Subsystem1 ==
  In1 : Inport
  Action Port : ActionPort  ActionPortLabel=elseif( u1 >= 1.715)
  LUT 1.72RR : Lookup_n-D  NumberOfTableDimensions=1  BreakpointsForDimension1=[428.7096;527.6572;623.7681;719.7739;815.4526;910.8868;1006.145;1101.276;1196.313;1291.279;1386.19;1481.059;1575.895;1670.704;1765.49;1860.259;1955.013]  Table=[400;500;600;700;800;900;1000;1100;1200;1300;1400;1500;1600;1700;1800;1900;2000]  InternalRulePriority=Speed  RndMeth=Simplest
  Out1 : Outport
  wires:
  In1/1 -> LUT 1.72RR/1
  LUT 1.72RR/1 -> Out1/1

== system LUT_kidney_25/If Action Subsystem6/If Action Subsystem2/If Action Subsystem7/If Action Subsystem10 ==
  In1 : Inport
  Action Port : ActionPort  ActionPortLabel=elseif( u1>= 1.705)
  LUT 1.71RR : Lookup_n-D  NumberOfTableDimensions=1  BreakpointsForDimension1=[428.7655;527.7212;623.8452;719.8698;815.5717;911.0324;1006.32;1101.482;1196.551;1291.55;1386.495;1481.399;1576.27;1671.115;1765.938;1860.743;1955.534]  Table=[400;500;600;700;800;900;1000;1100;1200;1300;1400;1500;1600;1700;1800;1900;2000]  InternalRulePriority=Speed  RndMeth=Simplest
  Out1 : Outport
  wires:
  In1/1 -> LUT 1.71RR/1
  LUT 1.71RR/1 -> Out1/1

== system LUT_kidney_25/If Action Subsystem6/If Action Subsystem2/If Action Subsystem7/If Action Subsystem2 ==
  In1 : Inport
  Action Port : ActionPort  ActionPortLabel=else
  LUT 1.70RR : Lookup_n-D  NumberOfTableDimensions=1  BreakpointsForDimension1=[428.8219;527.7861;623.9236;719.9675;815.6931;911.1807;1006.498;1101.691;1196.792;1291.825;1386.806;1481.745;1576.652;1671.533;1766.392;1861.235;1956.063]  Table=[400;500;600;700;800;900;1000;1100;1200;1300;1400;1500;1600;1700;1800;1900;2000]  InternalRulePriority=Speed  RndMeth=Simplest
  Out1 : Outport
  wires:
  In1/1 -> LUT 1.70RR/1
  LUT 1.70RR/1 -> Out1/1

== system LUT_kidney_25/If Action Subsystem6/If Action Subsystem2/If Action Subsystem7/If Action Subsystem3 ==
  In1 : Inport
  Action Port : ActionPort  ActionPortLabel=elseif( u1 >= 1.725)
  LUT 1.73RR : Lookup_n-D  NumberOfTableDimensions=1  BreakpointsForDimension1=[428.6543;527.5941;623.6922;719.6797;815.3357;910.744;1005.974;1101.075;1196.08;1291.013;1385.89;1480.725;1575.526;1670.299;1765.05;1859.783;1954.501]  Table=[400;500;600;700;800;900;1000;1100;1200;1300;1400;1500;1600;1700;1800;1900;2000]  InternalRulePriority=Speed  RndMeth=Simplest
  Out1 : Outport
  wires:
  In1/1 -> LUT 1.73RR/1
  LUT 1.73RR/1 -> Out1/1

== system LUT_kidney_25/If Action Subsystem6/If Action Subsystem2/If Action Subsystem7/If Action Subsystem4 ==
  In1 : Inport
  Action Port : ActionPort  ActionPortLabel=elseif( u1 >= 1.735)
  LUT 1.74RR : Lookup_n-D  NumberOfTableDimensions=1  BreakpointsForDimension1=[428.5995;527.5318;623.6176;719.5872;815.2211;910.6038;1005.806;1100.877;1195.85;1290.751;1385.596;1480.396;1575.163;1669.901;1764.617;1859.314;1953.996]  Table=[400;500;600;700;800;900;1000;1100;1200;1300;1400;1500;1600;1700;1800;1900;2000]  InternalRulePriority=Speed  RndMeth=Simplest
  Out1 : Outport
  wires:
  In1/1 -> LUT 1.74RR/1
  LUT 1.74RR/1 -> Out1/1

== system LUT_kidney_25/If Action Subsystem6/If Action Subsystem2/If Action Subsystem7/If Action Subsystem5 ==
  In1 : Inport
  Action Port : ActionPort  ActionPortLabel=elseif( u1 >= 1.755)
  LUT 1.76RR : Lookup_n-D  NumberOfTableDimensions=1  BreakpointsForDimension1=[428.4914;527.4097;623.4721;719.4073;814.9981;910.3313;1005.479;1100.491;1195.404;1290.241;1385.021;1479.755;1574.454;1669.124;1763.77;1858.398;1953.009]  Table=[400;500;600;700;800;900;1000;1100;1200;1300;1400;1500;1600;1700;1800;1900;2000]  InternalRulePriority=Speed  RndMeth=Simplest
  Out1 : Outport
  wires:
  In1/1 -> LUT 1.76RR/1
  LUT 1.76RR/1 -> Out1/1

== system LUT_kidney_25/If Action Subsystem6/If Action Subsystem2/If Action Subsystem7/If Action Subsystem6 ==
  In1 : Inport
  Action Port : ActionPort  ActionPortLabel=elseif( u1 >= 1.745)
  LUT 1.75RR : Lookup_n-D  NumberOfTableDimensions=1  BreakpointsForDimension1=[428.5452;527.4703;623.5442;719.4964;815.1085;910.4663;1005.641;1100.682;1195.625;1290.494;1385.306;1480.073;1574.805;1669.509;1764.19;1858.852;1953.499]  Table=[400;500;600;700;800;900;1000;1100;1200;1300;1400;1500;1600;1700;1800;1900;2000]  InternalRulePriority=Speed  RndMeth=Simplest
  Out1 : Outport
  wires:
  In1/1 -> LUT 1.75RR/1
  LUT 1.75RR/1 -> Out1/1

== system LUT_kidney_25/If Action Subsystem6/If Action Subsystem2/If Action Subsystem7/If Action Subsystem7 ==
  In1 : Inport
  Action Port : ActionPort  ActionPortLabel=elseif( u1 >= 1.765)
  LUT 1.77RR : Lookup_n-D  NumberOfTableDimensions=1  BreakpointsForDimension1=[428.4381;527.3498;623.4011;719.3198;814.8898;910.1988;1005.32;1100.304;1195.187;1289.993;1384.741;1479.443;1574.108;1668.744;1763.357;1857.95;1952.527]  Table=[400;500;600;700;800;900;1000;1100;1200;1300;1400;1500;1600;1700;1800;1900;2000]  InternalRulePriority=Speed  RndMeth=Simplest
  Out1 : Outport
  wires:
  In1/1 -> LUT 1.77RR/1
  LUT 1.77RR/1 -> Out1/1

== system LUT_kidney_25/If Action Subsystem6/If Action Subsystem2/If Action Subsystem7/If Action Subsystem8 ==
  In1 : Inport
  Action Port : ActionPort  ActionPortLabel=elseif(u1 >= 1.775)
  LUT 1.78RR : Lookup_n-D  NumberOfTableDimensions=1  BreakpointsForDimension1=[428.3854;527.2908;623.3312;719.2338;814.7834;910.0689;1005.164;1100.12;1194.973;1289.749;1384.465;1479.135;1573.768;1668.371;1762.95;1857.51;1952.053]  Table=[400;500;600;700;800;900;1000;1100;1200;1300;1400;1500;1600;1700;1800;1900;2000]  InternalRulePriority=Speed  RndMeth=Simplest
  Out1 : Outport
  wires:
  In1/1 -> LUT 1.78RR/1
  LUT 1.78RR/1 -> Out1/1

== system LUT_kidney_25/If Action Subsystem6/If Action Subsystem2/If Action Subsystem7/If Action Subsystem9 ==
  In1 : Inport
  Action Port : ActionPort  ActionPortLabel=if(u1 >= 1.785)
  LUT 1.79RR : Lookup_n-D  NumberOfTableDimensions=1  BreakpointsForDimension1=[428.3331;527.2325;623.2625;719.1494;814.6791;909.9413;1005.011;1099.939;1194.763;1289.509;1384.194;1478.833;1573.433;1668.004;1762.55;1857.076;1951.585]  Table=[400;500;600;700;800;900;1000;1100;1200;1300;1400;1500;1600;1700;1800;1900;2000]  InternalRulePriority=Speed  RndMeth=Simplest
  Out1 : Outport
  wires:
  In1/1 -> LUT 1.79RR/1
  LUT 1.79RR/1 -> Out1/1

== system LUT_kidney_25/If Action Subsystem6/If Action Subsystem2/If Action Subsystem8/If Action Subsystem1 ==
  In1 : Inport
  Action Port : ActionPort  ActionPortLabel=elseif( u1 >= 1.815)
  LUT 1.82RR : Lookup_n-D  NumberOfTableDimensions=1  BreakpointsForDimension1=[428.1791;527.062;623.063;718.9052;814.3776;909.5728;1004.568;1099.416;1194.156;1288.814;1383.409;1477.955;1572.461;1666.936;1761.386;1855.814;1950.225]  Table=[400;500;600;700;800;900;1000;1100;1200;1300;1400;1500;1600;1700;1800;1900;2000]  InternalRulePriority=Speed  RndMeth=Simplest
  Out1 : Outport
  wires:
  In1/1 -> LUT 1.82RR/1
  LUT 1.82RR/1 -> Out1/1

== system LUT_kidney_25/If Action Subsystem6/If Action Subsystem2/If Action Subsystem8/If Action Subsystem10 ==
  In1 : Inport
  Action Port : ActionPort  ActionPortLabel=elseif( u1>= 1.805)
  LUT 1.81RR : Lookup_n-D  NumberOfTableDimensions=1  BreakpointsForDimension1=[428.23;527.1181;623.1284;718.9851;814.4762;909.6933;1004.712;1099.587;1194.355;1289.042;1383.666;1478.242;1572.78;1667.286;1761.768;1856.228;1950.672]  Table=[400;500;600;700;800;900;1000;1100;1200;1300;1400;1500;1600;1700;1800;1900;2000]  InternalRulePriority=Speed  RndMeth=Simplest
  Out1 : Outport
  wires:
  In1/1 -> LUT 1.81RR/1
  LUT 1.81RR/1 -> Out1/1

== system LUT_kidney_25/If Action Subsystem6/If Action Subsystem2/If Action Subsystem8/If Action Subsystem2 ==
  In1 : Inport
  Action Port : ActionPort  ActionPortLabel=else
  LUT 1.80RR : Lookup_n-D  NumberOfTableDimensions=1  BreakpointsForDimension1=[428.2813;527.1749;623.1949;719.0665;814.5767;909.8162;1004.86;1099.762;1194.557;1289.273;1383.928;1478.535;1573.104;1667.642;1762.156;1856.649;1951.125]  Table=[400;500;600;700;800;900;1000;1100;1200;1300;1400;1500;1600;1700;1800;1900;2000]  InternalRulePriority=Speed  RndMeth=Simplest
  Out1 : Outport
  wires:
  In1/1 -> LUT 1.80RR/1
  LUT 1.80RR/1 -> Out1/1

== system LUT_kidney_25/If Action Subsystem6/If Action Subsystem2/If Action Subsystem8/If Action Subsystem3 ==
  In1 : Inport
  Action Port : ActionPort  ActionPortLabel=elseif( u1 >= 1.825)
  LUT 1.83RR : Lookup_n-D  NumberOfTableDimensions=1  BreakpointsForDimension1=[428.1288;527.0066;622.9986;718.8267;814.2808;909.4545;1004.425;1099.248;1193.961;1288.59;1383.156;1477.671;1572.147;1666.592;1761.01;1855.406;1949.785]  Table=[400;500;600;700;800;900;1000;1100;1200;1300;1400;1500;1600;1700;1800;1900;2000]  InternalRulePriority=Speed  RndMeth=Simplest
  Out1 : Outport
  wires:
  In1/1 -> LUT 1.83RR/1
  LUT 1.83RR/1 -> Out1/1

== system LUT_kidney_25/If Action Subsystem6/If Action Subsystem2/If Action Subsystem8/If Action Subsystem4 ==
  In1 : Inport
  Action Port : ActionPort  ActionPortLabel=elseif( u1 >= 1.835)
  LUT 1.84RR : Lookup_n-D  NumberOfTableDimensions=1  BreakpointsForDimension1=[428.0788;526.952;622.9353;718.7496;814.1859;909.3385;1004.286;1099.083;1193.769;1288.37;1382.907;1477.393;1571.839;1666.252;1760.639;1855.005;1949.352]  Table=[400;500;600;700;800;900;1000;1100;1200;1300;1400;1500;1600;1700;1800;1900;2000]  InternalRulePriority=Speed  RndMeth=Simplest
  Out1 : Outport
  wires:
  In1/1 -> LUT 1.84RR/1
  LUT 1.84RR/1 -> Out1/1

== system LUT_kidney_25/If Action Subsystem6/If Action Subsystem2/If Action Subsystem8/If Action Subsystem5 ==
  In1 : Inport
  Action Port : ActionPort  ActionPortLabel=elseif( u1 >= 1.855)
  LUT 1.86RR : Lookup_n-D  NumberOfTableDimensions=1  BreakpointsForDimension1=[427.9803;526.8447;622.8116;718.5995;814.0012;909.1129;1004.014;1098.762;1193.395;1287.942;1382.422;1476.85;1571.236;1665.59;1759.916;1854.22;1948.505]  Table=[400;500;600;700;800;900;1000;1100;1200;1300;1400;1500;1600;1700;1800;1900;2000]  InternalRulePriority=Speed  RndMeth=Simplest
  Out1 : Outport
  wires:
  In1/1 -> LUT 1.86RR/1
  LUT 1.86RR/1 -> Out1/1

== system LUT_kidney_25/If Action Subsystem6/If Action Subsystem2/If Action Subsystem8/If Action Subsystem6 ==
  In1 : Inport
  Action Port : ActionPort  ActionPortLabel=elseif( u1 >= 1.845)
  LUT 1.85RR : Lookup_n-D  NumberOfTableDimensions=1  BreakpointsForDimension1=[428.0294;526.898;622.8729;718.6739;814.0927;909.2246;1004.149;1098.921;1193.58;1288.154;1382.662;1477.119;1571.535;1665.918;1760.275;1854.609;1948.925]  Table=[400;500;600;700;800;900;1000;1100;1200;1300;1400;1500;1600;1700;1800;1900;2000]  InternalRulePriority=Speed  RndMeth=Simplest
  Out1 : Outport
  wires:
  In1/1 -> LUT 1.85RR/1
  LUT 1.85RR/1 -> Out1/1

== system LUT_kidney_25/If Action Subsystem6/If Action Subsystem2/If Action Subsystem8/If Action Subsystem7 ==
  In1 : Inport
  Action Port : ActionPort  ActionPortLabel=elseif( u1 >= 1.865)
  LUT 1.87RR : Lookup_n-D  NumberOfTableDimensions=1  BreakpointsForDimension1=[427.9318;526.7921;622.7512;718.5265;813.9115;909.0032;1003.882;1098.605;1193.213;1287.733;1382.185;1476.585;1570.942;1665.266;1759.562;1853.836;1948.091]  Table=[400;500;600;700;800;900;1000;1100;1200;1300;1400;1500;1600;1700;1800;1900;2000]  InternalRulePriority=Speed  RndMeth=Simplest
  Out1 : Outport
  wires:
  In1/1 -> LUT 1.87RR/1
  LUT 1.87RR/1 -> Out1/1

== system LUT_kidney_25/If Action Subsystem6/If Action Subsystem2/If Action Subsystem8/If Action Subsystem8 ==
  In1 : Inport
  Action Port : ActionPort  ActionPortLabel=elseif(u1 >= 1.875)
  LUT 1.88RR : Lookup_n-D  NumberOfTableDimensions=1  BreakpointsForDimension1=[427.8836;526.7401;622.6917;718.4547;813.8234;908.8956;1003.753;1098.452;1193.034;1287.528;1381.953;1476.324;1570.653;1664.948;1759.214;1853.458;1947.683]  Table=[400;500;600;700;800;900;1000;1100;1200;1300;1400;1500;1600;1700;1800;1900;2000]  InternalRulePriority=Speed  RndMeth=Simplest
  Out1 : Outport
  wires:
  In1/1 -> LUT 1.88RR/1
  LUT 1.88RR/1 -> Out1/1

== system LUT_kidney_25/If Action Subsystem6/If Action Subsystem2/If Action Subsystem8/If Action Subsystem9 ==
  In1 : Inport
  Action Port : ActionPort  ActionPortLabel=if(u1 >= 1.885)
  LUT 1.89RR : Lookup_n-D  NumberOfTableDimensions=1  BreakpointsForDimension1=[427.8359;526.6887;622.6332;718.3843;813.737;908.79;1003.625;1098.301;1192.859;1287.326;1381.724;1476.067;1570.368;1664.634;1758.872;1853.086;1947.281]  Table=[400;500;600;700;800;900;1000;1100;1200;1300;1400;1500;1600;1700;1800;1900;2000]  InternalRulePriority=Speed  RndMeth=Simplest
  Out1 : Outport
  wires:
  In1/1 -> LUT 1.89RR/1
  LUT 1.89RR/1 -> Out1/1

== system LUT_kidney_25/If Action Subsystem6/If Action Subsystem2/If Action Subsystem9/If Action Subsystem1 ==
  In1 : Inport
  Action Port : ActionPort  ActionPortLabel=elseif( u1 >= 1.915)
  LUT 1.92RR : Lookup_n-D  NumberOfTableDimensions=1  BreakpointsForDimension1=[427.6953;526.5384;622.4631;718.1803;813.4872;908.485;1003.258;1097.865;1192.35;1286.741;1381.06;1475.323;1569.541;1663.723;1757.875;1852.003;1946.111]  Table=[400;500;600;700;800;900;1000;1100;1200;1300;1400;1500;1600;1700;1800;1900;2000]  InternalRulePriority=Speed  RndMeth=Simplest
  Out1 : Outport
  wires:
  In1/1 -> LUT 1.92RR/1
  LUT 1.92RR/1 -> Out1/1

== system LUT_kidney_25/If Action Subsystem6/If Action Subsystem2/If Action Subsystem9/If Action Subsystem10 ==
  In1 : Inport
  Action Port : ActionPort  ActionPortLabel=if(u1 >= 1.995)
  LUT 2.00RR : Lookup_n-D  NumberOfTableDimensions=1  BreakpointsForDimension1=[427.3379;526.1631;622.0465;717.6871;812.8866;907.752;1002.373;1096.814;1191.119;1285.323;1379.446;1473.508;1567.52;1661.492;1755.431;1849.344;1943.234]  Table=[400;500;600;700;800;900;1000;1100;1200;1300;1400;1500;1600;1700;1800;1900;2000]  InternalRulePriority=Speed  RndMeth=Simplest
  Out1 : Outport
  wires:
  In1/1 -> LUT 2.00RR/1
  LUT 2.00RR/1 -> Out1/1
